simulink model "modelo_mecanico_doble_pendulo"  (R2022b)
settings: Solver=VariableStepAuto  StartTime=0.0  StopTime=10.0  MaxStep=t_muestreo  RelTol=1e-3
values from neighbouring files (symbols this model uses):
  g = 9.81    [mecanico_doble_pendulo.m]
  in_theta1 = 0    [mecanico_doble_pendulo.m]
  in_theta1_d1 = 0    [mecanico_doble_pendulo.m]
  in_theta2 = (7*pi)/36    (= 0.610865238198)    [mecanico_doble_pendulo.m]
  in_theta2_d1 = 0    [mecanico_doble_pendulo.m]
  l1 = .3    (= 0.3)    [mecanico_doble_pendulo.m]
  l2 = .25    (= 0.25)    [mecanico_doble_pendulo.m]
  m1 = .2    (= 0.2)    [mecanico_doble_pendulo.m]
  m2 = .1    (= 0.1)    [mecanico_doble_pendulo.m]
settings Model: Creator=frayg  LastModifiedBy=frayg

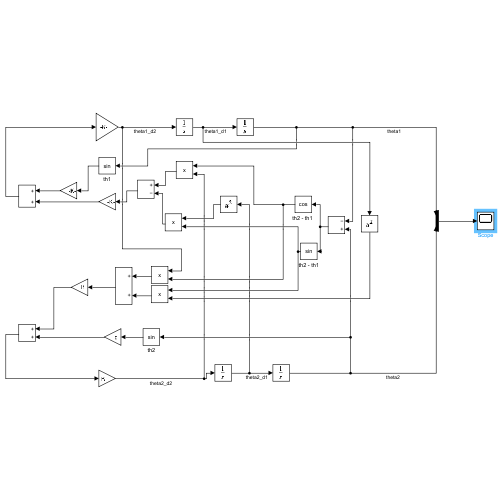
[thumbnail: Simulink's stored preview of the top-level diagram]
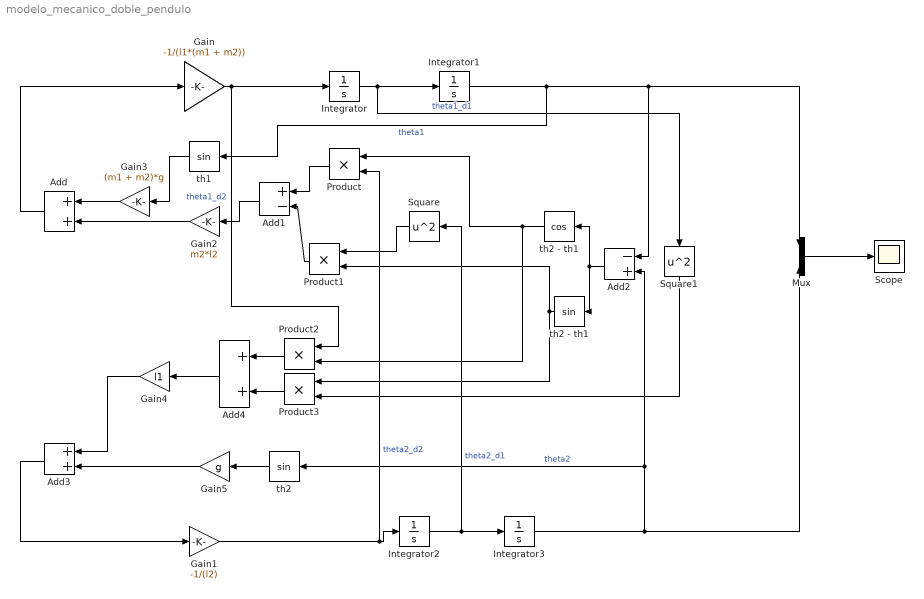
== system modelo_mecanico_doble_pendulo ==
  Add : Sum
  Add1 : Sum  Inputs=+-
  Add2 : Sum  Inputs=-+
  Add3 : Sum
  Add4 : Sum
  Gain : Gain  Gain=-1/(l1*(m1 + m2))
  Gain1 : Gain  Gain=-1/(l2)
  Gain2 : Gain  Gain=m2*l2
  Gain3 : Gain  Gain=(m1 + m2)*g
  Gain4 : Gain  Gain=l1
  Gain5 : Gain  Gain=g
  Integrator : Integrator  InitialCondition=in_theta1_d1
  Integrator1 : Integrator  InitialCondition=in_theta1
  Integrator2 : Integrator  InitialCondition=in_theta2_d1
  Integrator3 : Integrator  InitialCondition=in_theta2
  Mux : Mux  Inputs=2
  Product{,1..3} (4 alike) : Product
  Scope : Scope
  Square : Math  Operator=square
  Square1 : Math  Operator=square
  th1 : Trigonometry
  th2 : Trigonometry
  th2 - th1 : Trigonometry
  "th2 - th1 " : Trigonometry  Operator=cos
  wires:
  Gain/1 -> Product2/1, Integrator/1  "theta1_d2"
  Integrator/1 -> Square1/1, Integrator1/1  "theta1_d1"
  Integrator1/1 -> th1/1, Add2/1, Mux/1  "theta1"
  Gain1/1 -> Product/2, Integrator2/1  "theta2_d2"
  Integrator2/1 -> Square/1, Integrator3/1  "theta2_d1"
  Integrator3/1 -> th2/1, Add2/2, Mux/2  "theta2"
  Add/1 -> Gain/1
  Add1/1 -> Gain2/1
  Product/1 -> Add1/1
  Add2/1 -> "th2 - th1 "/1, th2 - th1/1
  "th2 - th1 "/1 -> Product2/2, Product/1
  Product1/1 -> Add1/2
  Square/1 -> Product1/1
  th2 - th1/1 -> Product3/1, Product1/2
  Gain2/1 -> Add/2
  Gain3/1 -> Add/1
  th1/1 -> Gain3/1
  Add3/1 -> Gain1/1
  Gain4/1 -> Add3/1
  Add4/1 -> Gain4/1
  Product2/1 -> Add4/1
  Product3/1 -> Add4/2
  Square1/1 -> Product3/2
  Gain5/1 -> Add3/2
  th2/1 -> Gain5/1
  Mux/1 -> Scope/1
